simulink model "PID_Controller"  (R2020a)
settings: Solver=VariableStepAuto  StartTime=0.0  StopTime=10.0  RelTol=1e-3
undefined symbols (not defined in the file): kd, ki, kp
settings Model: Creator=sreeram  LastModifiedBy=sreeram
settings DataIOCC: SaveOutput=off  SaveTime=off

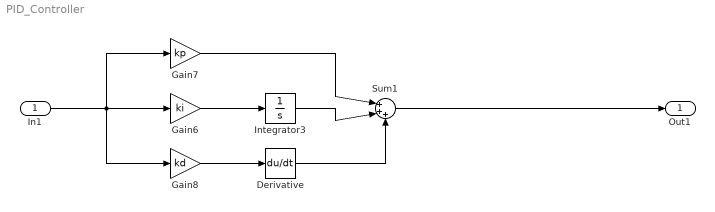
== system PID_Controller ==
  In1 : Inport  OutDataTypeStr=double  PortDimensions=1  SampleTime=0
  Derivative : Derivative
  Gain6 : Gain  Gain=ki
  Gain7 : Gain  Gain=kp
  Gain8 : Gain  Gain=kd
  Integrator3 : Integrator
  Sum1 : Sum  Inputs=|+++
  Out1 : Outport  OutDataTypeStr=double  PortDimensions=1  SampleTime=0
  wires:
  Sum1/1 -> Out1/1
  Gain6/1 -> Integrator3/1
  In1/1 -> Gain6/1, Gain7/1, Gain8/1
  Integrator3/1 -> Sum1/2
  Gain7/1 -> Sum1/1
  Gain8/1 -> Derivative/1
  Derivative/1 -> Sum1/3
